simulink library "utility"  (R2024b)
settings: Solver=VariableStepAuto  StartTime=0.0  StopTime=10.0  RelTol=1e-3
undefined symbols (not defined in the file or in its folder): DiscIntNeverNeededParam
libraries: $bdroot x1, simulink x1
settings Model: Creator=loq  LastModifiedBy=loq

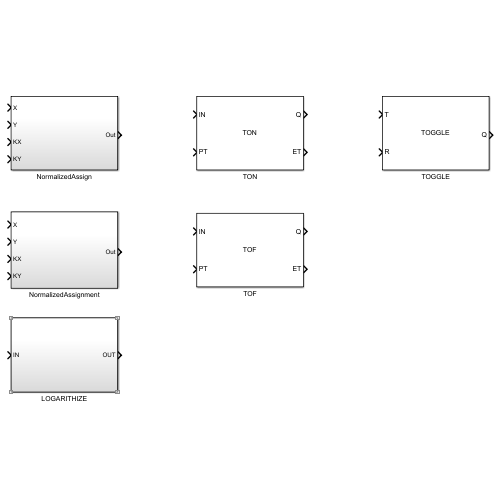
[thumbnail: Simulink's stored preview of the top-level diagram]
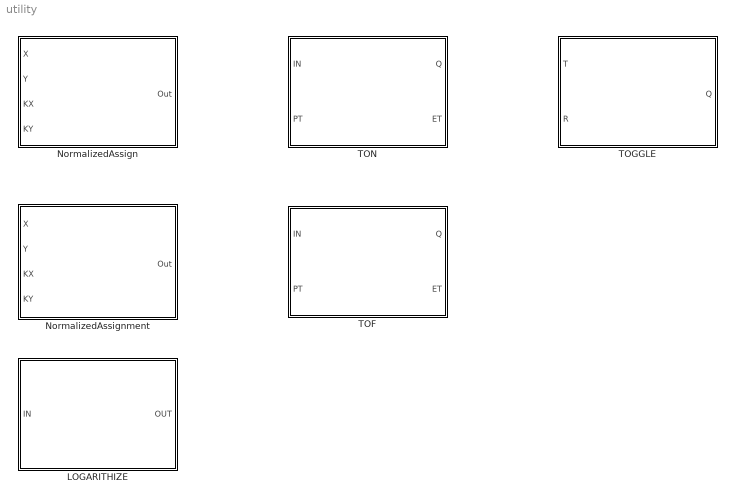
== system utility ==
  LOGARITHIZE : Subsystem
  NormalizedAssign : Subsystem
  NormalizedAssignment : Subsystem
  TOF : Subsystem
      mask Display:
      | disp('TOF');
      | port_label('output', 1, 'Q');
      | port_label('output', 2, 'ET');
      | port_label('input', 1, 'IN');
      | port_label('input', 2, 'PT');
  TOGGLE : Subsystem
      mask Display:
      | disp('TOGGLE');
      | port_label('output', 1, 'Q');
      | port_label('input', 1, 'T');
      | port_label('input', 2, 'R');
  TON : Subsystem
      mask Display:
      | disp('TON');
      | port_label('output', 1, 'Q');
      | port_label('output', 2, 'ET');
      | port_label('input', 1, 'IN');
      | port_label('input', 2, 'PT');

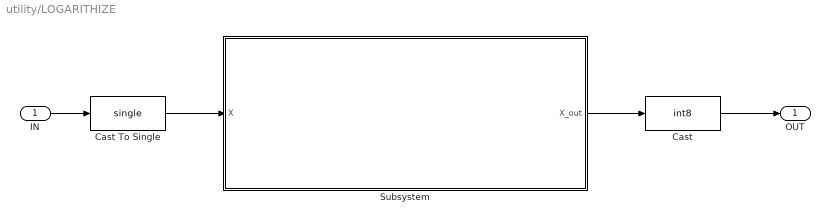
== system utility/LOGARITHIZE ==
  IN : Inport  OutDataTypeStr=int8
  Cast : DataTypeConversion  OutDataTypeStr=int8  RndMeth=Floor
  Cast To Single : DataTypeConversion  OutDataTypeStr=single  SaturateOnIntegerOverflow=off  RndMeth=Floor
  Subsystem : Subsystem
  OUT : Outport  OutDataTypeStr=int8
  wires:
  Subsystem/1(X_out) -> Cast/1
  Cast To Single/1 -> Subsystem/1(X)
  IN/1 -> Cast To Single/1
  Cast/1 -> OUT/1

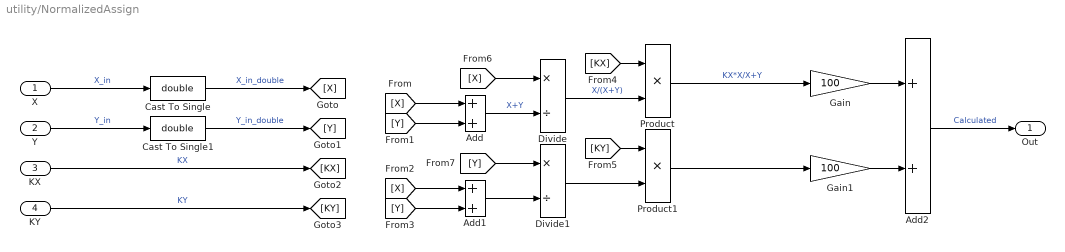
== system utility/NormalizedAssign ==
  X : Inport  OutDataTypeStr=int8
  Y : Inport  Port=2  OutDataTypeStr=int8
  KX : Inport  Port=3  OutDataTypeStr=double
  KY : Inport  Port=4  OutDataTypeStr=double
  Add : Sum
  Add1 : Sum
  Add2 : Sum  OutDataTypeStr=double
  Cast To Single : DataTypeConversion  OutDataTypeStr=double  SaturateOnIntegerOverflow=off  RndMeth=Floor
  Cast To Single1 : DataTypeConversion  OutDataTypeStr=double  SaturateOnIntegerOverflow=off  RndMeth=Floor
  Divide : Product  Inputs=*/
  Divide1 : Product  Inputs=*/
  Gain : Gain  Gain=100
  Gain1 : Gain  Gain=100
  Product : Product
  Product1 : Product
  Out : Outport  OutDataTypeStr=double
  wires:
  Add1/1 -> Divide1/2
  Divide1/1 -> Product1/2
  Divide/1 -> Product/2  "X/(X+Y)"
  Add/1 -> Divide/2  "X+Y"
  [X] -> Add/1
  [Y] -> Add/2
  [Y] -> Add1/2
  [X] -> Add1/1
  [KX] -> Product/1
  [KY] -> Product1/1
  [X] -> Divide/1
  [Y] -> Divide1/1
  Product/1 -> Gain/1  "KX*X/X+Y"
  Product1/1 -> Gain1/1
  X/1 -> Cast To Single/1  "X_in"
  Y/1 -> Cast To Single1/1  "Y_in"
  KX/1 -> [KX]  "KX"
  KY/1 -> [KY]  "KY"
  Add2/1 -> Out/1  "Calculated"
  Cast To Single/1 -> [X]  "X_in_double"
  Cast To Single1/1 -> [Y]  "Y_in_double"
  Gain/1 -> Add2/1
  Gain1/1 -> Add2/2

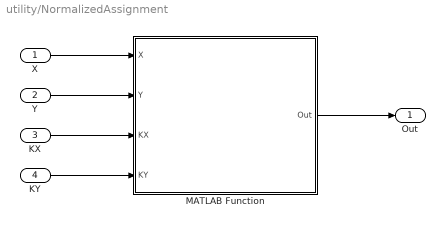
== system utility/NormalizedAssignment ==
  X : Inport  OutDataTypeStr=int8
  Y : Inport  Port=2  OutDataTypeStr=int8
  KX : Inport  Port=3  OutDataTypeStr=int8
  KY : Inport  Port=4  OutDataTypeStr=int8
  MATLAB Function : MATLAB Function  TreatAsAtomicUnit=on
  Out : Outport  OutDataTypeStr=int8
  wires:
  MATLAB Function/1(Out) -> Out/1
  X/1 -> MATLAB Function/1(X)
  Y/1 -> MATLAB Function/2(Y)
  KX/1 -> MATLAB Function/3(KX)
  KY/1 -> MATLAB Function/4(KY)

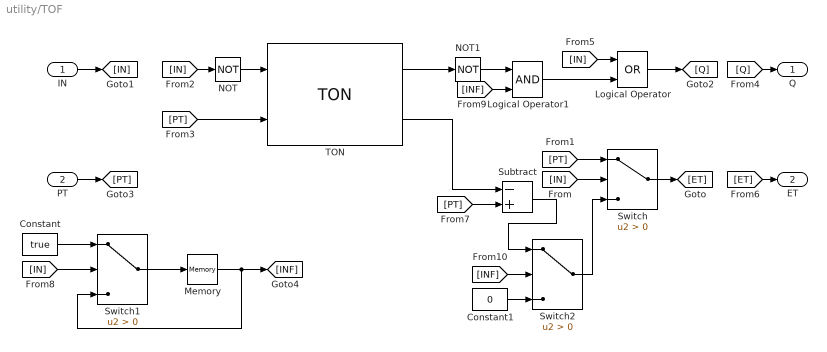
== system utility/TOF ==
  IN : Inport  OutDataTypeStr=boolean
  PT : Inport  Port=2  OutDataTypeStr=single
  Constant : Constant  Value=true
  Constant1 : Constant  Value=0  OutDataTypeStr=single
  Logical Operator : Logic  Operator=OR  AllPortsSameDT=off  OutDataTypeStr=boolean
  Logical Operator1 : Logic  AllPortsSameDT=off  OutDataTypeStr=boolean
  Memory : Memory  InitialCondition=false
  NOT : Logic  Operator=NOT  IconShape=distinctive  AllPortsSameDT=off  OutDataTypeStr=boolean
  NOT1 : Logic  Operator=NOT  IconShape=distinctive  AllPortsSameDT=off  OutDataTypeStr=boolean
  Subtract : Sum  Inputs=-+
  Switch : Switch  Criteria=u2 > Threshold  SaturateOnIntegerOverflow=off  InputSameDT=off
  Switch1 : Switch  Criteria=u2 > Threshold  SaturateOnIntegerOverflow=off  InputSameDT=off
  Switch2 : Switch  Criteria=u2 > Threshold  SaturateOnIntegerOverflow=off  InputSameDT=off
  TON : $bdroot/TON  SystemSampleTime=-1  VariantActivationTime=update diagram  AllowFlexibleInterface=on  Latency=0  AutoFrameSizeCalculation=off
  Q : Outport  OutDataTypeStr=boolean
  ET : Outport  Port=2  OutDataTypeStr=single
  wires:
  [Q] -> Q/1
  IN/1 -> [IN]
  [ET] -> ET/1
  PT/1 -> [PT]
  [IN] -> Switch/2
  Switch/1 -> [ET]
  [PT] -> Switch/1
  [IN] -> NOT/1
  NOT/1 -> TON/1
  [PT] -> TON/2
  [IN] -> Logical Operator/1
  Logical Operator/1 -> [Q]
  TON/1 -> NOT1/1
  [PT] -> Subtract/2
  TON/2 -> Subtract/1
  [IN] -> Switch1/2
  Memory/1 -> [INF], Switch1/3
  Constant/1 -> Switch1/1
  Switch1/1 -> Memory/1
  NOT1/1 -> Logical Operator1/1
  Logical Operator1/1 -> Logical Operator/2
  [INF] -> Logical Operator1/2
  [INF] -> Switch2/2
  Switch2/1 -> Switch/3
  Subtract/1 -> Switch2/1
  Constant1/1 -> Switch2/3

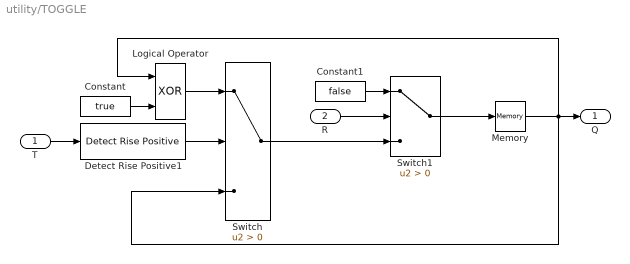
== system utility/TOGGLE ==
  T : Inport  OutDataTypeStr=boolean
  R : Inport  Port=2  OutDataTypeStr=boolean
  Constant : Constant  Value=true  OutDataTypeStr=boolean
  Constant1 : Constant  Value=false  OutDataTypeStr=boolean
  Detect Rise Positive1 : simulink/Logic and Bit Operations/Detect Rise Positive  vinit=0  OutDataTypeStr=boolean
  Logical Operator : Logic  Operator=XOR  AllPortsSameDT=off  OutDataTypeStr=boolean
  Memory : Memory
  Switch : Switch  Criteria=u2 > Threshold  OutDataTypeStr=boolean  SaturateOnIntegerOverflow=off  InputSameDT=off
  Switch1 : Switch  Criteria=u2 > Threshold  SaturateOnIntegerOverflow=off  InputSameDT=off
  Q : Outport  OutDataTypeStr=boolean
  wires:
  R/1 -> Switch1/2
  Constant1/1 -> Switch1/1
  Switch/1 -> Switch1/3
  Logical Operator/1 -> Switch/1
  Constant/1 -> Logical Operator/2
  Memory/1 -> Q/1, Switch/3, Logical Operator/1
  Detect Rise Positive1/1 -> Switch/2
  Switch1/1 -> Memory/1
  T/1 -> Detect Rise Positive1/1

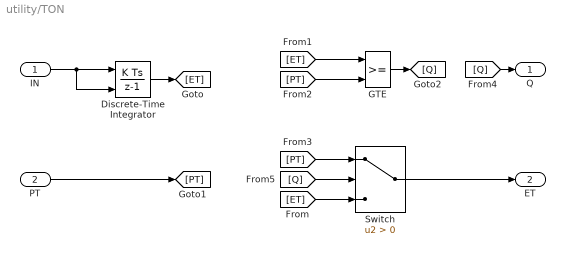
== system utility/TON ==
  IN : Inport  OutDataTypeStr=boolean
  PT : Inport  Port=2  OutDataTypeStr=single
  Discrete-Time Integrator : DiscreteIntegrator  ExternalReset=falling  SampleTime=-1  OutDataTypeStr=single  ICPrevOutput=DiscIntNeverNeededParam  ICPrevScaledInput=DiscIntNeverNeededParam
  GTE : RelationalOperator  OutDataTypeStr=boolean  RndMeth=Simplest  InputSameDT=off
  Switch : Switch  Criteria=u2 > Threshold  SaturateOnIntegerOverflow=off  InputSameDT=off
  Q : Outport  OutDataTypeStr=boolean
  ET : Outport  Port=2  OutDataTypeStr=single
  wires:
  IN/1 -> Discrete-Time Integrator/2, Discrete-Time Integrator/1
  Discrete-Time Integrator/1 -> [ET]
  PT/1 -> [PT]
  [ET] -> GTE/1
  [PT] -> GTE/2
  Switch/1 -> ET/1
  [ET] -> Switch/3
  [PT] -> Switch/1
  GTE/1 -> [Q]
  [Q] -> Q/1
  [Q] -> Switch/2

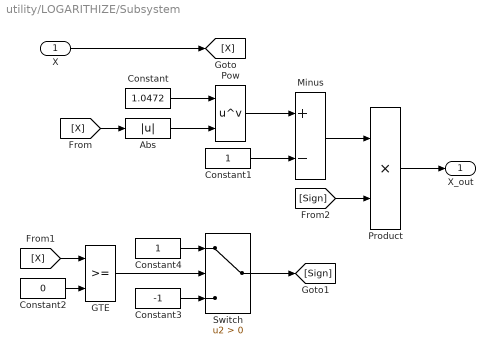
== system utility/LOGARITHIZE/Subsystem ==
  X : Inport  OutDataTypeStr=single
  Abs : Abs  SaturateOnIntegerOverflow=off
  Constant : Constant  Value=1.0472  OutDataTypeStr=single
  Constant1 : Constant  OutDataTypeStr=single
  Constant2 : Constant  Value=0  OutDataTypeStr=single
  Constant3 : Constant  Value=-1  OutDataTypeStr=single
  Constant4 : Constant  OutDataTypeStr=single
  GTE : RelationalOperator  OutDataTypeStr=boolean  RndMeth=Simplest  InputSameDT=off
  Minus : Sum  Inputs=+-
  Pow : Math  Operator=pow  SignedPower=on  RndMeth=Zero
  Product : Product
  Switch : Switch  Criteria=u2 > Threshold  SaturateOnIntegerOverflow=off  InputSameDT=off
  X_out : Outport  OutDataTypeStr=single
  wires:
  Abs/1 -> Pow/2
  [X] -> Abs/1
  Constant/1 -> Pow/1
  Pow/1 -> Minus/1
  Constant1/1 -> Minus/2
  Constant2/1 -> GTE/2
  [X] -> GTE/1
  GTE/1 -> Switch/2
  Constant3/1 -> Switch/3
  Constant4/1 -> Switch/1
  Switch/1 -> [Sign]
  Minus/1 -> Product/1
  [Sign] -> Product/2
  Product/1 -> X_out/1
  X/1 -> [X]

== matlab function utility/NormalizedAssignment/MATLAB Function ==
  data: X input; Out output; Y input; KX input; KY input
function Out = NormalizedAssignment(X, Y, KX, KY)

    max_val = 100; 
    x = double(X);
    y = double(Y);
    kx = double(KX);
    ky = double(KY);

    if abs(x) + abs(y) < 1e-6
        Out = int8(0);
        return
    end

    projection = (kx * x) + (ky * y);

    projection = max(min(projection, max_val), -max_val);

    Out = int8(round(projection));
end
